simulink model "mymodel"  (R2019b)
settings: Solver=ode45  StartTime=0.0  StopTime=20  RelTol=1e-3
settings Model: Creator=don  LastModifiedBy=don
settings DataIOCC: TimeSaveName=mytime

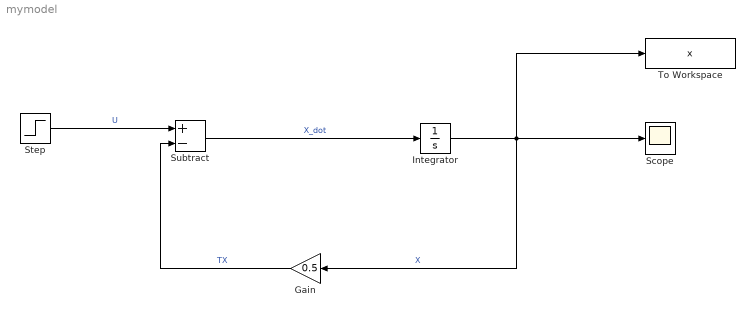
== system mymodel ==
  Gain : Gain  Gain=0.5
  Integrator : Integrator
  Scope : Scope
  Step : Step  After=10  SampleTime=0
  Subtract : Sum  Inputs=+-
  To Workspace : ToWorkspace  VariableName=x  SampleTime=-1
  wires:
  Step/1 -> Subtract/1  "U"
  Subtract/1 -> Integrator/1  "X_dot"
  Integrator/1 -> Gain/1, Scope/1, To Workspace/1  "X"
  Gain/1 -> Subtract/2  "TX"
